simulink model "LQGI_Nonlinear"  (R2024b)
settings: Solver=VariableStepAuto  StartTime=0.0  StopTime=10.0  RelTol=1e-10
values from neighbouring files (symbols this model uses):
  A = [0, 0, 0, 1, 0, 0;        0, 0, 0, 0, 1, 0;        0, 0, 0, 0, 0, 1;        0, 0, -(M^2*g*h^2*r^2)/(2*I*I_y + 2*I*M*h^2 + I_y*M*r^2 + 2*I_y*m*r^2 + 2*M*h^2*m*r^2), 0, 0, 0;        0, 0, 0, 0, 0, 0;        0, 0, (2*g*h*M^2*r^2 + 4*g*h*m*M*r^2 + 4*I*g*h*M)/(4*I*I_y + 4*I*M*h^2 + 2*I_y*M*r^2 + 4*I_y*m*r^2 + 4*M*h^2*m*r^2), 0, 0, 0]    [Controllability.m]    (also in LQGI_Calculations.m = [0, 0, 0, 1, 0, 0;        0, 0, 0, 0, 1, 0;        0, 0, 0, ; LQR.m = [0, 0, 0, 1, 0, 0;        0, 0, 0, 0, 1, 0;        0, 0, 0, ; Observability.m; Pole_Placement.m = [0, 0, 0, 1, 0, 0;        0, 0, 0, 0, 1, 0;        0, 0, 0, )
  B = [0, 0;       0, 0;       0, 0;       (r*(M*h^2 + M*r*h + I_y))/(2*I*I_y + 2*I*M*h^2 + I_y*M*r^2 + 2*I_y*m*r^2 + 2*M*h^2*m*r^2), (r*(M*h^2 + M*r*h + I_y))/(2*I*I_y + 2*I*M*h^2 + I_y*M*r^2 + 2*I_y*m*r^2 + 2*M*h^2*m*r^2);     -(a*r)/(2*m*a^2*r^2 + 2*I*a^2 + I_z*r^2), (a*r)/(2*m*a^2*r^2 + 2*I*a^2 + I_z*r^2);     -(4*I + 2*M*r^2 + 4*m*r^2 + 2*M*h*r)/(4*I*I_y + 4*I*M*h^2 + 2*I_y*M*r^2 + 4*I_y*m*r^2 + 4* ...(+117 chars)    [Controllability.m]    (also in LQGI_Calculations.m = [0, 0;        0, 0;        0, 0;        (r*(M*h^2 + M*r*h + ; LQR.m = [0, 0;       0, 0;       0, 0;       (r*(M*h^2 + M*r*h + I_y; Observability.m; Pole_Placement.m = [0, 0;       0, 0;       0, 0;       (r*(M*h^2 + M*r*h + I_y)
  C_Kalman = C(1:3, :)    [LQGI_Calculations.m]
  D_Kalman = D(1:3, :)    [LQGI_Calculations.m]
  K_I = lqi(sys_k,  Q, R, 0)    [LQGI_Calculations.m]
  psi_ref = pi/4    (= 0.785398163397)    [LQGI_Calculations.m]
  rho_ref = 2    [LQGI_Calculations.m]
undefined symbols (not defined in the file or in its folder): Continuous, Time
libraries: simulink x1, ctrlSharedLib x1
settings Model: Creator=appenteng.adjepong  LastModifiedBy=appenteng.adjepong

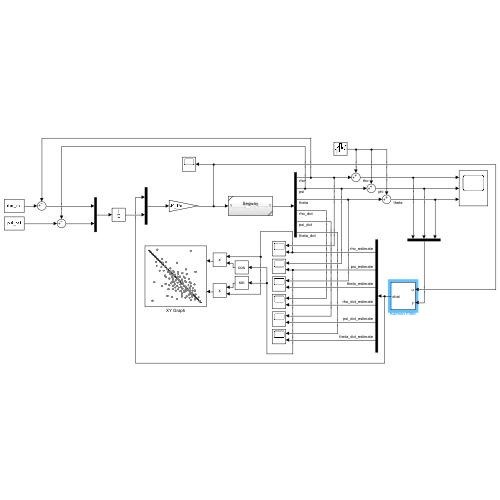
[thumbnail: Simulink's stored preview of the top-level diagram]
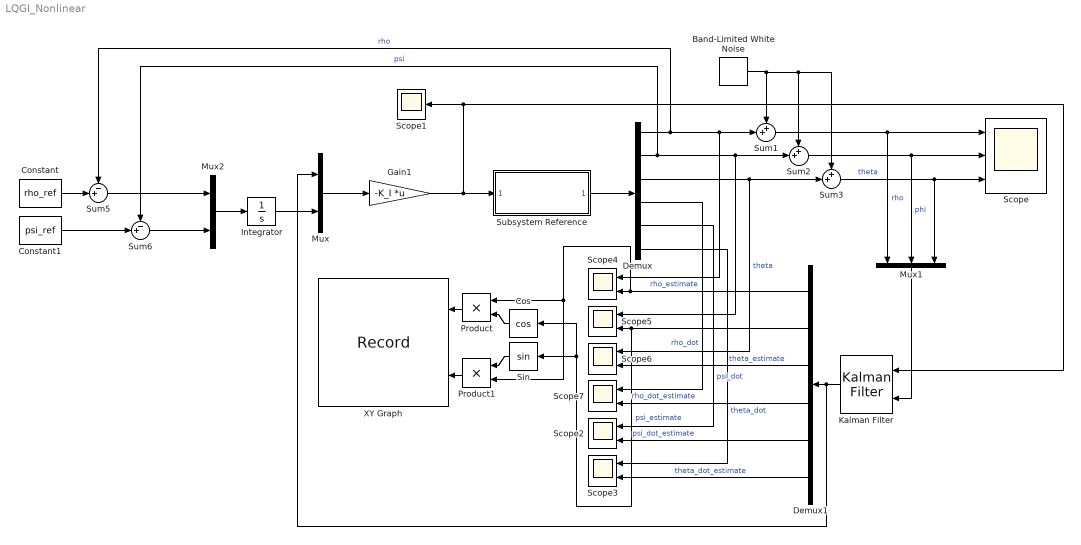
== system LQGI_Nonlinear ==
  Band-Limited White Noise : simulink/Sources/Band-Limited White Noise  Cov=10e-4  Ts=0.1  seed=[23341]
  Constant : Constant  Value=rho_ref
  Constant1 : Constant  Value=psi_ref
  Cos : Trigonometry  Operator=cos
  Demux : Demux  Outputs=6
  Demux1 : Demux  Outputs=6
  Gain1 : Gain  Gain=-K_I  Multiplication=Matrix(K*u)
  Integrator : Integrator
  Kalman Filter : ctrlSharedLib/Kalman Filter  TimeDomain=Continuous-Time  UseCurrentEstimator=on  ModelSource=LTI State-Space Variable  ModelSourceVariable=ss(A, B, C_Kalman, D_Kalman)  A=0.95  B=1  C=1  D=0  NumberOfStates=1  NumberOfInputs=1  NumberOfOutputs=1  InitialEstimateSource=Dialog  X0=0  P0=10  UseK=off  UseGH=on  NumberOfProcessNoiseInputs=1  G=B  TimeInvariantG=on  H=0  TimeInvariantH=on  Q=1e-6  TimeInvariantQ=on  R=1e-2  TimeInvariantR=on  N=0  TimeInvariantN=on  AddInputPort=on  AddEnablePort=off  OutputEstimatedY=off  OutputP=off  Ts=-1
  Mux : Mux  Inputs=2
  Mux1 : Mux  Inputs=3
  Mux2 : Mux  Inputs=2
  Product : Product
  Product1 : Product
  Scope : Scope  NumInputPorts=3
  Scope1 : Scope
  Scope{2..7} (6 alike) : Scope  NumInputPorts=2
  Sin : Trigonometry
  Subsystem Reference : Subsystem  ReferencedSubsystem=Segway
  Sum1 : Sum  Inputs=++|
  Sum2 : Sum  Inputs=++|
  Sum3 : Sum  Inputs=++|
  Sum5 : Sum  Inputs=-+|
  Sum6 : Sum  Inputs=-+|
  XY Graph : Record  FileSettingsInternal="{\"entries\":[{\"content\":{\"excelSettings\":{\"content\":{},\"type\":\"Streamout.ExcelSettings\"}},\"type\":\"Streamout.FileSettingStorage\",\"uuid\":\"\"}],\"packageUris\":[\"http:\\/\\/schema.mathworks.com\\/mf0\\/streamout_blocks\\/R2020a\"],\"version\":\"1.0\"}"  Layout=[1 1]  SignalsInternal="{\"entries\":[{\"content\":{\"signals\":[{\"content\":{\"blockPath\":[],\"dimensions\":[1],\"domain\":\"\",\"lineColor\":\"#a2142f\",\"lineWidth\":2,\"plots\":[ 1 ],\"port\":1,\"sid\":[\"\"],\"signalID\":1,\"signalName\":\"Product\"},\"type\":\"RecordBlkView.Signal\",\"uuid\":\"\"},{\"content\":{\"blockPath\":[],\"dimensions\":[1],\"domain\":\"\",\"lineColor\":\"#139fff\",\"lineWidth\":2,\"plots\":[ 1 ],\"port\":2,\"sid\":[\"\"],\"signalID\":2,\"signalName\":\"Product1\"},\"type\":\"RecordBlkView.Signal\",\"uuid\":\"\"}]},\"type\":\"RecordBlkView.InputSignals\",\"uuid\":\"\"}],\"packageUris\":[\"http:\\/\\/schema.mathworks.com\\/mf0\\/streamout_blocks\\/R2020a\"],\"version\":\"1.0\"}"  VisualizationBindings="{\"xyplotplugin\":{\"info\":[{\"series\":[{\"bindingParametersList\":[{\"parameter\":\"X-Axis\",\"signalID\":1,\"signalName\":\"Product\"},{\"parameter\":\"Y-Axis\",\"signalID\":2,\"signalName\":\"Product1\"}],\"seriesID\":0},{\"bindingParametersList\":[{\"parameter\":\"X-Axis\",\"signalID\":1,\"signalName\":\"Product\"}],\"seriesID\":1}],\"subplotID\":1}]}}"  CompatibilityTag=XY
  wires:
  Product1/1 -> XY Graph/2
  Sin/1 -> Product1/1
  Demux1/3 -> Scope6/2  "theta_estimate"
  Mux2/1 -> Integrator/1
  Integrator/1 -> Mux/2
  Demux/2 -> Scope5/1, Sum2/2, Sum6/1  "psi"
  Mux/1 -> Gain1/1
  Demux1/5 -> Scope2/2  "psi_dot_estimate"
  Demux1/6 -> Scope3/2  "theta_dot_estimate"
  Sum1/1 -> Scope/1, Mux1/1  "rho"
  Cos/1 -> Product/2
  Demux/5 -> Scope2/1  "psi_dot"
  Gain1/1 -> Subsystem Reference/1, Scope1/1, Kalman Filter/1
  Demux/1 -> Scope4/1, Sum1/2, Sum5/1  "rho"
  Demux1/4 -> Scope7/2  "rho_dot_estimate"
  Sum3/1 -> Scope/3, Mux1/3  "theta"
  Kalman Filter/1 -> Mux/1, Demux1/1
  Demux1/1 -> Product/1, Product1/2, Scope4/2  "rho_estimate"
  Constant/1 -> Sum5/2
  Product/1 -> XY Graph/1
  Demux/3 -> Scope6/1, Sum3/2  "theta"
  Demux1/2 -> Sin/1, Cos/1, Scope5/2  "psi_estimate"
  Sum2/1 -> Scope/2, Mux1/2  "phi"
  Demux/6 -> Scope3/1  "theta_dot"
  Subsystem Reference/1 -> Demux/1
  Band-Limited White Noise/1 -> Sum3/1, Sum2/1, Sum1/1
  Mux1/1 -> Kalman Filter/2
  Constant1/1 -> Sum6/2
  Sum5/1 -> Mux2/1
  Demux/4 -> Scope7/1  "rho_dot"
  Sum6/1 -> Mux2/2
